simulink model "Simulink_Program_June26 1"  (R2023b)
settings: Solver=VariableStepAuto  StartTime=0.0  StopTime=1  FixedStep=0.001  RelTol=1e-3
libraries: fl_lib x11, nesl_utility x9, ee_lib x7
settings Model: Creator=romul  LastModifiedBy=mcmas

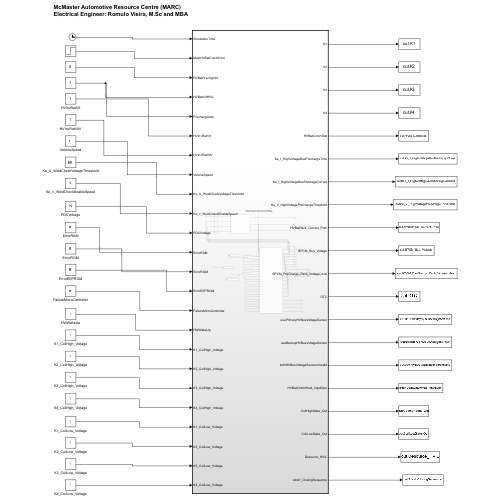
[thumbnail: Simulink's stored preview of the top-level diagram]
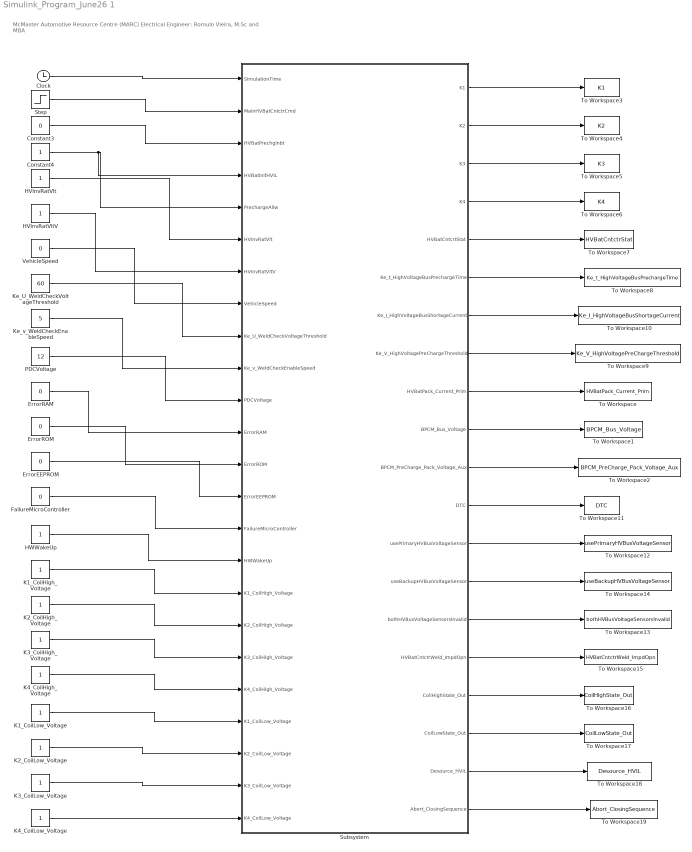
== system Simulink_Program_June26 1 ==
  note: McMaster Automotive Resource Centre (MARC)
      | Electrical Engineer: Romulo Vieira, M.Sc and MBA
  Clock : Clock
  Constant3 : Constant  Value=0
  Constant4 : Constant
  ErrorEEPROM : Constant  Value=0
  ErrorRAM : Constant  Value=0
  ErrorROM : Constant  Value=0
  FailureMicroController : Constant  Value=0
  HVInvRatVlt : Constant
  HVInvRatVltV : Constant
  HWWakeUp : Constant
  K1_CoilHigh_Voltage : Constant
  K1_CoilLow_Voltage : Constant
  K2_CoilHigh_Voltage : Constant
  K2_CoilLow_Voltage : Constant
  K3_CoilHigh_Voltage : Constant
  K3_CoilLow_Voltage : Constant
  K4_CoilHigh_Voltage : Constant
  K4_CoilLow_Voltage : Constant
  Ke_U_WeldCheckVoltageThreshold : Constant  Value=60
  Ke_v_WeldCheckEnableSpeed : Constant  Value=5
  PDCVoltage : Constant  Value=12
  Step : Step  Time=0.5  SampleTime=0.001
  Subsystem : Subsystem  TreatAsAtomicUnit=on
  To Workspace : ToWorkspace  VariableName=HVBatPack_Current_Prim  SampleTime=-1
  To Workspace1 : ToWorkspace  VariableName=BPCM_Bus_Voltage  SampleTime=-1
  To Workspace10 : ToWorkspace  VariableName=Ke_I_HighVoltageBusShortageCurrent  SampleTime=-1
  To Workspace11 : ToWorkspace  VariableName=DTC  SaveFormat=Timeseries  SampleTime=-1
  To Workspace12 : ToWorkspace  VariableName=usePrimaryHVBusVoltageSensor  SaveFormat=Timeseries  SampleTime=-1
  To Workspace13 : ToWorkspace  VariableName=bothHVBusVoltageSensorsInvalid  SaveFormat=Timeseries  SampleTime=-1
  To Workspace14 : ToWorkspace  VariableName=useBackupHVBusVoltageSensor  SaveFormat=Timeseries  SampleTime=-1
  To Workspace15 : ToWorkspace  VariableName=HVBatCntctrWeld_ImpdOpn  SaveFormat=Timeseries  SampleTime=-1
  To Workspace16 : ToWorkspace  VariableName=CoilHighState_Out  SaveFormat=Timeseries  SampleTime=-1
  To Workspace17 : ToWorkspace  VariableName=CoilLowState_Out  SaveFormat=Timeseries  SampleTime=-1
  To Workspace18 : ToWorkspace  VariableName=Desource_HVIL  SaveFormat=Timeseries  SampleTime=-1
  To Workspace19 : ToWorkspace  VariableName=Abort_ClosingSequence  SaveFormat=Timeseries  SampleTime=-1
  To Workspace2 : ToWorkspace  VariableName=BPCM_PreCharge_Pack_Voltage_Aux  SampleTime=-1
  To Workspace3 : ToWorkspace  VariableName=K1  SampleTime=-1
  To Workspace4 : ToWorkspace  VariableName=K2  SampleTime=-1
  To Workspace5 : ToWorkspace  VariableName=K3  SampleTime=-1
  To Workspace6 : ToWorkspace  VariableName=K4  SampleTime=-1
  To Workspace7 : ToWorkspace  VariableName=HVBatCntctrStat  SampleTime=-1
  To Workspace8 : ToWorkspace  VariableName=Ke_t_HighVoltageBusPrechargeTime  SampleTime=-1
  To Workspace9 : ToWorkspace  VariableName=Ke_V_HighVoltagePreChargeThreshold  SampleTime=-1
  VehicleSpeed : Constant  Value=0
  wires:
  Subsystem/3(K3) -> To Workspace5/1
  HVInvRatVltV/1 -> Subsystem/7(HVInvRatVltV)
  Subsystem/15(bothHVBusVoltageSensorsInvalid) -> To Workspace13/1
  Subsystem/6(Ke_t_HighVoltageBusPrechargeTime) -> To Workspace8/1
  HVInvRatVlt/1 -> Subsystem/6(HVInvRatVlt)
  Subsystem/18(CoilLowState_Out) -> To Workspace17/1
  Clock/1 -> Subsystem/1(SimulationTime)
  Constant4/1 -> Subsystem/4(HVBatInitHVIL), Subsystem/5(PrechargeAllw)
  Subsystem/8(Ke_V_HighVoltagePreChargeThreshold) -> To Workspace9/1
  K3_CoilHigh_Voltage/1 -> Subsystem/19(K3_CoilHigh_Voltage)
  Constant3/1 -> Subsystem/3(HVBatPrechgInbt)
  Step/1 -> Subsystem/2(MainHVBatCntctrCmd)
  Ke_U_WeldCheckVoltageThreshold/1 -> Subsystem/9(Ke_U_WeldCheckVoltageThreshold)
  Subsystem/16(HVBatCntctrWeld_ImpdOpn) -> To Workspace15/1
  VehicleSpeed/1 -> Subsystem/8(VehicleSpeed)
  K1_CoilLow_Voltage/1 -> Subsystem/21(K1_CoilLow_Voltage)
  Ke_v_WeldCheckEnableSpeed/1 -> Subsystem/10(Ke_v_WeldCheckEnableSpeed)
  HWWakeUp/1 -> Subsystem/16(HWWakeUp)
  PDCVoltage/1 -> Subsystem/11(PDCVoltage)
  ErrorRAM/1 -> Subsystem/12(ErrorRAM)
  ErrorROM/1 -> Subsystem/13(ErrorROM)
  ErrorEEPROM/1 -> Subsystem/14(ErrorEEPROM)
  FailureMicroController/1 -> Subsystem/15(FailureMicroController)
  Subsystem/1(K1) -> To Workspace3/1
  K1_CoilHigh_Voltage/1 -> Subsystem/17(K1_CoilHigh_Voltage)
  K2_CoilHigh_Voltage/1 -> Subsystem/18(K2_CoilHigh_Voltage)
  K4_CoilHigh_Voltage/1 -> Subsystem/20(K4_CoilHigh_Voltage)
  K2_CoilLow_Voltage/1 -> Subsystem/22(K2_CoilLow_Voltage)
  Subsystem/7(Ke_I_HighVoltageBusShortageCurrent) -> To Workspace10/1
  K3_CoilLow_Voltage/1 -> Subsystem/23(K3_CoilLow_Voltage)
  K4_CoilLow_Voltage/1 -> Subsystem/24(K4_CoilLow_Voltage)
  Subsystem/2(K2) -> To Workspace4/1
  Subsystem/4(K4) -> To Workspace6/1
  Subsystem/5(HVBatCntcrtStat) -> To Workspace7/1
  Subsystem/9(HVBatPack_Current_Prim) -> To Workspace/1
  Subsystem/10(BPCM_Bus_Voltage) -> To Workspace1/1
  Subsystem/14(useBackupHVBusVoltageSensor) -> To Workspace14/1
  Subsystem/12(DTC) -> To Workspace11/1
  Subsystem/11(BPCM_PreCharge_Pack_Voltage_Aux) -> To Workspace2/1
  Subsystem/13(usePrimaryHVBusVoltageSensor) -> To Workspace12/1
  Subsystem/17(CoilHighState_Out) -> To Workspace16/1
  Subsystem/19(Desource_HVIL) -> To Workspace18/1
  Subsystem/20(Abort_ClosingSequence) -> To Workspace19/1

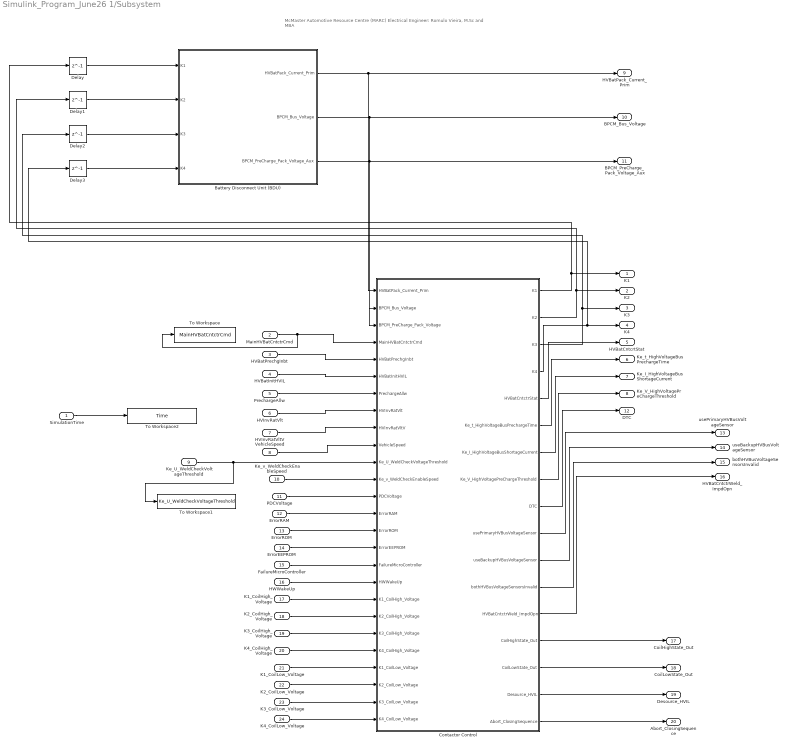
== system Simulink_Program_June26 1/Subsystem ==
  note: McMaster Automotive Resource Centre (MARC)
      | Electrical Engineer: Romulo Vieira, M.Sc and MBA
  SimulationTime : Inport
  MainHVBatCntctrCmd : Inport  Port=2
  HVBatPrechgInbt : Inport  Port=3
  HVBatInitHVIL : Inport  Port=4
  PrechargeAllw : Inport  Port=5
  HVInvRatVlt : Inport  Port=6
  HVInvRatVltV : Inport  Port=7
  VehicleSpeed : Inport  Port=8
  Ke_U_WeldCheckVoltageThreshold : Inport  Port=9
  Ke_v_WeldCheckEnableSpeed : Inport  Port=10
  PDCVoltage : Inport  Port=11
  ErrorRAM : Inport  Port=12
  ErrorROM : Inport  Port=13
  ErrorEEPROM : Inport  Port=14
  FailureMicroController : Inport  Port=15
  HWWakeUp : Inport  Port=16
  K1_CoilHigh_Voltage : Inport  Port=17
  K2_CoilHigh_Voltage : Inport  Port=18
  K3_CoilHigh_Voltage : Inport  Port=19
  K4_CoilHigh_Voltage : Inport  Port=20
  K1_CoilLow_Voltage : Inport  Port=21
  K2_CoilLow_Voltage : Inport  Port=22
  K3_CoilLow_Voltage : Inport  Port=23
  K4_CoilLow_Voltage : Inport  Port=24
  Battery Disconnect Unit (BDU) : Subsystem  TreatAsAtomicUnit=on
  Contactor Control : Subsystem  TreatAsAtomicUnit=on  SystemSampleTime=0.001
  Delay{,1..3} (4 alike) : Delay  DelayLength=1
  To Workspace : ToWorkspace  VariableName=MainHVBatCntctrCmd  SampleTime=-1
  To Workspace1 : ToWorkspace  VariableName=Ke_U_WeldCheckVoltageThreshold  SampleTime=-1
  To Workspace2 : ToWorkspace  VariableName=Time  SampleTime=0.001
  K1 : Outport
  K2 : Outport  Port=2
  K3 : Outport  Port=3
  K4 : Outport  Port=4
  HVBatCntcrtStat : Outport  Port=5
  Ke_t_HighVoltageBusPrechargeTime : Outport  Port=6
  Ke_I_HighVoltageBusShortageCurrent : Outport  Port=7
  Ke_V_HighVoltagePreChargeThreshold : Outport  Port=8
  HVBatPack_Current_Prim : Outport  Port=9
  BPCM_Bus_Voltage : Outport  Port=10
  BPCM_PreCharge_Pack_Voltage_Aux : Outport  Port=11
  DTC : Outport  Port=12
  usePrimaryHVBusVoltageSensor : Outport  Port=13
  useBackupHVBusVoltageSensor : Outport  Port=14
  bothHVBusVoltageSensorsInvalid : Outport  Port=15
  HVBatCntctrWeld_ImpdOpn : Outport  Port=16
  CoilHighState_Out : Outport  Port=17
  CoilLowState_Out : Outport  Port=18
  Desource_HVIL : Outport  Port=19
  Abort_ClosingSequence : Outport  Port=20
  wires:
  Battery Disconnect Unit (BDU)/1(HVBatPack_Current_Prim) -> Contactor Control/1(HVBatPack_Current_Prim), HVBatPack_Current_Prim/1
  Battery Disconnect Unit (BDU)/2(BPCM_Bus_Voltage) -> BPCM_Bus_Voltage/1, Contactor Control/2(BPCM_Bus_Voltage)
  MainHVBatCntctrCmd/1 -> To Workspace/1, Contactor Control/4(MainHVBatCntctrCmd)
  HVBatPrechgInbt/1 -> Contactor Control/5(HVBatPrechgInbt)
  HVBatInitHVIL/1 -> Contactor Control/6(HVBatInitHVIL)
  PrechargeAllw/1 -> Contactor Control/7(PrechargeAllw)
  Contactor Control/1(K1) -> Delay/1, K1/1
  Contactor Control/2(K2) -> Delay1/1, K2/1
  Contactor Control/3(K3) -> Delay2/1, K3/1
  Contactor Control/4(K4) -> Delay3/1, K4/1
  Contactor Control/5(HVBatCntctrStat) -> HVBatCntcrtStat/1
  Contactor Control/6(Ke_t_HighVoltageBusPrechargeTime) -> Ke_t_HighVoltageBusPrechargeTime/1
  Contactor Control/7(Ke_I_HighVoltageBusShortageCurrent) -> Ke_I_HighVoltageBusShortageCurrent/1
  Contactor Control/8(Ke_V_HighVoltagePreChargeThreshold) -> Ke_V_HighVoltagePreChargeThreshold/1
  Battery Disconnect Unit (BDU)/3(BPCM_PreCharge_Pack_Voltage_Aux) -> BPCM_PreCharge_Pack_Voltage_Aux/1, Contactor Control/3(BPCM_PreCharge_Pack_Voltage)
  Delay/1 -> Battery Disconnect Unit (BDU)/1(K1)
  Delay1/1 -> Battery Disconnect Unit (BDU)/2(K2)
  Delay2/1 -> Battery Disconnect Unit (BDU)/3(K3)
  Delay3/1 -> Battery Disconnect Unit (BDU)/4(K4)
  Contactor Control/9(DTC) -> DTC/1
  HVInvRatVlt/1 -> Contactor Control/8(HVInvRatVlt)
  HVInvRatVltV/1 -> Contactor Control/9(HVInvRatVltV)
  Contactor Control/10(usePrimaryHVBusVoltageSensor) -> usePrimaryHVBusVoltageSensor/1
  Contactor Control/11(useBackupHVBusVoltageSensor) -> useBackupHVBusVoltageSensor/1
  Contactor Control/12(bothHVBusVoltageSensorsInvalid) -> bothHVBusVoltageSensorsInvalid/1
  Contactor Control/13(HVBatCntctrWeld_ImpdOpn) -> HVBatCntctrWeld_ImpdOpn/1
  VehicleSpeed/1 -> Contactor Control/10(VehicleSpeed)
  Ke_U_WeldCheckVoltageThreshold/1 -> To Workspace1/1, Contactor Control/11(Ke_U_WeldCheckVoltageThreshold)
  Ke_v_WeldCheckEnableSpeed/1 -> Contactor Control/12(Ke_v_WeldCheckEnableSpeed)
  ErrorRAM/1 -> Contactor Control/14(ErrorRAM)
  ErrorROM/1 -> Contactor Control/15(ErrorROM)
  PDCVoltage/1 -> Contactor Control/13(PDCVoltage)
  FailureMicroController/1 -> Contactor Control/17(FailureMicroController)
  HWWakeUp/1 -> Contactor Control/18(HWWakeUp)
  ErrorEEPROM/1 -> Contactor Control/16(ErrorEEPROM)
  SimulationTime/1 -> To Workspace2/1
  K1_CoilHigh_Voltage/1 -> Contactor Control/19(K1_CoilHigh_Voltage)
  K2_CoilHigh_Voltage/1 -> Contactor Control/20(K2_CoilHigh_Voltage)
  K4_CoilHigh_Voltage/1 -> Contactor Control/22(K4_CoilHigh_Voltage)
  K3_CoilHigh_Voltage/1 -> Contactor Control/21(K3_CoilHigh_Voltage)
  K2_CoilLow_Voltage/1 -> Contactor Control/24(K2_CoilLow_Voltage)
  K1_CoilLow_Voltage/1 -> Contactor Control/23(K1_CoilLow_Voltage)
  K4_CoilLow_Voltage/1 -> Contactor Control/26(K4_CoilLow_Voltage)
  K3_CoilLow_Voltage/1 -> Contactor Control/25(K3_CoilLow_Voltage)
  Contactor Control/14(CoilHighState_Out) -> CoilHighState_Out/1
  Contactor Control/15(CoilLowState_Out) -> CoilLowState_Out/1
  Contactor Control/16(Desource_HVIL) -> Desource_HVIL/1
  Contactor Control/17(Abort_ClosingSequence) -> Abort_ClosingSequence/1

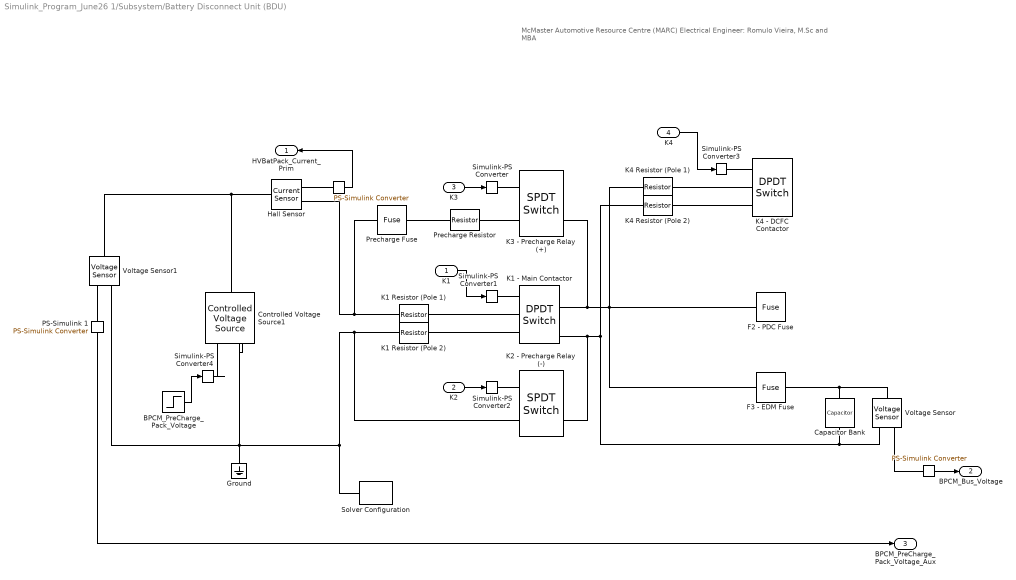
== system Simulink_Program_June26 1/Subsystem/Battery Disconnect Unit (BDU) ==
  note: McMaster Automotive Resource Centre (MARC)
      | Electrical Engineer: Romulo Vieira, M.Sc and MBA
  K1 : Inport
  K2 : Inport  Port=2
  K3 : Inport  Port=3
  K4 : Inport  Port=4
  "   " : nesl_utility/PS-Simulink Converter  PhysicalDomain=network_engine_domain  SubClassName=ps_output  LeftPortType=input  RightPortType=output  PseudoPeriodic=off  Frequencies=[]  VectorFormat=inherit  Unit=inherit  AffineConversion=off
  " " : nesl_utility/PS-Simulink Converter  PhysicalDomain=network_engine_domain  SubClassName=ps_output  LeftPortType=input  RightPortType=output  PseudoPeriodic=off  Frequencies=[]  VectorFormat=inherit  Unit=inherit  AffineConversion=off
  BPCM_PreCharge_Pack_Voltage : Step  Time=0  After=450  SampleTime=0.001
  Capacitor Bank : fl_lib/Electrical/Electrical Elements/Capacitor  c=750e-6 F  r=1e-6 Ohm  g=0 1/Ohm  i_specify=off  i_priority=None  i=0 A  i_nominal_specify=off  i_nominal_unit=A  i_nominal_value=1  v_specify=off  v_priority=None  v=0 V  v_nominal_specify=off  v_nominal_unit=V  v_nominal_value=1  vc_specify=on  vc_priority=High  vc=0 V  vc_nominal_specify=off  vc_nominal_unit=V  vc_nominal_value=1
  Controlled Voltage Source1 : fl_lib/Electrical/Electrical Sources/Controlled Voltage Source
  F2 - PDC Fuse : ee_lib/Switches & Breakers/Fuse  prm=1  I_rated=125 A  melt_margin=1  T_fuse=0 s  I2t=1 A^2*s  I_vec=[1.9, 2, 2.5, 30] A  t_vec=[10000, 1, .3, .001] s  R_closed=0.01 Ohm  G_open=1e-8 1/Ohm  exposemeasurement=ee.enum.exposemeasurement.hidden
      settings: InternalSimscapePortConfiguration="{\"Bottom\":[],\"Left\":[{\"id\":\"p\",\"label\":\"\",\"type\":\"foundation.electrical.electrical\"}],\"Right\":[{\"id\":\"n\",\"label\":\"\",\"type\":\"foundation.electrical.electrical\"}],\"Top\":[]}"
  F3 - EDM Fuse : ee_lib/Switches & Breakers/Fuse  prm=1  I_rated=600 A  melt_margin=1  T_fuse=0 s  I2t=1 A^2*s  I_vec=[1.9, 2, 2.5, 30] A  t_vec=[10000, 1, .3, .001] s  R_closed=0.01 Ohm  G_open=1e-8 1/Ohm  exposemeasurement=ee.enum.exposemeasurement.hidden
      settings: InternalSimscapePortConfiguration="{\"Bottom\":[],\"Left\":[{\"id\":\"p\",\"label\":\"\",\"type\":\"foundation.electrical.electrical\"}],\"Right\":[{\"id\":\"n\",\"label\":\"\",\"type\":\"foundation.electrical.electrical\"}],\"Top\":[]}"
  Ground : fl_lib/Electrical/Electrical Elements/Electrical Reference
  Hall Sensor : fl_lib/Electrical/Electrical Sensors/Current Sensor
  K1 - Main Contactor : ee_lib/Switches & Breakers/DPDT Switch  R_closed=0.01 Ohm  G_open=1e-6 S  Threshold=0.5 V  Width=0 V  model_dynamics=0  t_on=1e-3 s  t_off=1e-3 s  initial_vT=0 V
      settings: InternalSimscapePortConfiguration="{\"Bottom\":[],\"Left\":[{\"id\":\"vT\",\"label\":\"vT\",\"type\":\"input\"},{\"id\":\"p1\",\"label\":\"\",\"type\":\"foundation.electrical.electrical\"},{\"id\":\"p2\",\"label\":\"\",\"type\":\"foundation.electrical.electrical\"}],\"Right\":[{\"id\":\"n11\",\"label\":\"\",\"type\":\"foundation.electrical.electrical\"},{\"id\":\"n12\",\"label\":\"\",\"type\":\"foundation.electrical.electrical\"},{\"id\":\"n21\",\"label\":\"\",\"type\":\"foundation.electrical.electrical\"},{\"id\":\"n22\",\"label\":\"\",\"type\":\"foundation.electrical.electrical\"}],\"Top\":[]}"
  K1 Resistor (Pole 1) : fl_lib/Electrical/Electrical Elements/Resistor  R=0.0003 Ohm  i_specify=off  i_priority=None  i=0 A  i_nominal_specify=off  i_nominal_unit=A  i_nominal_value=1  v_specify=off  v_priority=None  v=0 V  v_nominal_specify=off  v_nominal_unit=V  v_nominal_value=1
  K1 Resistor (Pole 2) : fl_lib/Electrical/Electrical Elements/Resistor  R=0.0003 Ohm  i_specify=off  i_priority=None  i=0 A  i_nominal_specify=off  i_nominal_unit=A  i_nominal_value=1  v_specify=off  v_priority=None  v=0 V  v_nominal_specify=off  v_nominal_unit=V  v_nominal_value=1
  K2 - Precharge Relay (-) : ee_lib/Switches & Breakers/SPDT Switch  R_closed=0.01 Ohm  G_open=1e-6 S  Threshold=0.5 V  Width=0 V  model_dynamics=0  t_on=1e-3 s  t_off=1e-3 s  initial_vT=0 V
  K3 - Precharge Relay (+) : ee_lib/Switches & Breakers/SPDT Switch  R_closed=0.01 Ohm  G_open=1e-6 S  Threshold=0.5 V  Width=0 V  model_dynamics=0  t_on=1e-3 s  t_off=1e-3 s  initial_vT=0 V
  K4 - DCFC Contactor : ee_lib/Switches & Breakers/DPDT Switch  R_closed=0.01 Ohm  G_open=1e-6 S  Threshold=0.5 V  Width=0 V  model_dynamics=0  t_on=1e-3 s  t_off=1e-3 s  initial_vT=0 V
      settings: InternalSimscapePortConfiguration="{\"Bottom\":[],\"Left\":[{\"id\":\"vT\",\"label\":\"vT\",\"type\":\"input\"},{\"id\":\"p1\",\"label\":\"\",\"type\":\"foundation.electrical.electrical\"},{\"id\":\"p2\",\"label\":\"\",\"type\":\"foundation.electrical.electrical\"}],\"Right\":[{\"id\":\"n11\",\"label\":\"\",\"type\":\"foundation.electrical.electrical\"},{\"id\":\"n12\",\"label\":\"\",\"type\":\"foundation.electrical.electrical\"},{\"id\":\"n21\",\"label\":\"\",\"type\":\"foundation.electrical.electrical\"},{\"id\":\"n22\",\"label\":\"\",\"type\":\"foundation.electrical.electrical\"}],\"Top\":[]}"
  K4 Resistor (Pole 1) : fl_lib/Electrical/Electrical Elements/Resistor  R=0.0003 Ohm  i_specify=off  i_priority=None  i=0 A  i_nominal_specify=off  i_nominal_unit=A  i_nominal_value=1  v_specify=off  v_priority=None  v=0 V  v_nominal_specify=off  v_nominal_unit=V  v_nominal_value=1
  K4 Resistor (Pole 2) : fl_lib/Electrical/Electrical Elements/Resistor  R=0.0003 Ohm  i_specify=off  i_priority=None  i=0 A  i_nominal_specify=off  i_nominal_unit=A  i_nominal_value=1  v_specify=off  v_priority=None  v=0 V  v_nominal_specify=off  v_nominal_unit=V  v_nominal_value=1
  PS-Simulink 1 : nesl_utility/PS-Simulink Converter  PhysicalDomain=network_engine_domain  SubClassName=ps_output  LeftPortType=input  RightPortType=output  PseudoPeriodic=off  Frequencies=[]  VectorFormat=inherit  Unit=inherit  AffineConversion=off
  Precharge Fuse : ee_lib/Switches & Breakers/Fuse  prm=1  I_rated=600 A  melt_margin=1  T_fuse=0 s  I2t=1 A^2*s  I_vec=[1.9, 2, 2.5, 30] A  t_vec=[10000, 1, .3, .001] s  R_closed=0.01 Ohm  G_open=1e-8 1/Ohm  exposemeasurement=ee.enum.exposemeasurement.hidden
      settings: InternalSimscapePortConfiguration="{\"Bottom\":[],\"Left\":[{\"id\":\"p\",\"label\":\"\",\"type\":\"foundation.electrical.electrical\"}],\"Right\":[{\"id\":\"n\",\"label\":\"\",\"type\":\"foundation.electrical.electrical\"}],\"Top\":[]}"
  Precharge Resistor : fl_lib/Electrical/Electrical Elements/Resistor  R=25 Ohm  i_specify=off  i_priority=None  i=0 A  i_nominal_specify=off  i_nominal_unit=A  i_nominal_value=1  v_specify=off  v_priority=None  v=0 V  v_nominal_specify=off  v_nominal_unit=V  v_nominal_value=1
  Simulink-PS Converter{,1..3} (4 alike) : nesl_utility/Simulink-PS Converter  PhysicalDomain=network_engine_domain  SubClassName=ps_input  LeftPortType=input  RightPortType=output  PseudoPeriodic=off  Frequencies=[]  NoiseDistribution=none  NoiseParameters=[]  Unit=1  AffineConversion=off  FilteringAndDerivatives=provide  SimscapeFilterOrder=1  InputFilterTimeConstant=0.001  UdotUserProvided=0
  Simulink-PS Converter4 : nesl_utility/Simulink-PS Converter  PhysicalDomain=network_engine_domain  SubClassName=ps_input  LeftPortType=input  RightPortType=output  PseudoPeriodic=off  Frequencies=[]  NoiseDistribution=none  NoiseParameters=[]  Unit=1  AffineConversion=off  FilteringAndDerivatives=filter  SimscapeFilterOrder=1  InputFilterTimeConstant=0.0000001  UdotUserProvided=0
  Solver Configuration : nesl_utility/Solver Configuration  PhysicalDomain=network_engine_domain  SubClassName=solver  LeftPortType=input  RightPortType=generic  Tones=[]  Harmonics=[]  SimulateNoise=off  Profile=off  UseLocalSampling=off  EnableSwitchedLinearOptims=on  FrequencyDomain=off  UseCCode=off  RelTol=0.001  AbsTol=0.001  MinStep=1e-09  ToWorkspace=off  RevertToSquareIcSolve=off  NumHomotopyIterations=100  PhasorMode=off  PhasorModeNumHarmonics=1  ConsistencySolver=NEWTON_XTOL_AFTER_FTOL  IndexReductionMethod=DerivativeReplacement  DoDC=off  ResidualTolerance=1e-09  ConsistencyTolSource=GLOBAL  ConsistencyAbsTol=0.001  ConsistencyRelTol=0.001  ConsistencyTolFactor=0.001  UseLocalSolver=off  LocalSolverChoice=NE_BACKWARD_EULER_ADVANCER  ResolveIndetEquations=on  FunctionEvalNumThread=1  LocalSolverSampleTime=0.001  DoFixedCost=off  MaxNonlinIter=3  MaxModeIter=2  ComputeImpulses=off  ImpulseIterations=2  LinearAlgebra=auto  LinearAlgebraNumThread=0  EquationFormulation=NE_TIME_EF  DelaysMemoryBudget=1024  AutomaticFiltering=on  FilteringTimeConstant=0.001  PartitionStorageMethod=AS_NEEDED  PartitionMemoryBudget=1024  PartitionMethod=ROBUST  MultibodyUseLocalSolver=off  MultibodyLocalSolverChoice=ODE1  MultibodyLocalSolverSampleTime=0.001
  Voltage Sensor : fl_lib/Electrical/Electrical Sensors/Voltage Sensor
  Voltage Sensor1 : fl_lib/Electrical/Electrical Sensors/Voltage Sensor
  HVBatPack_Current_Prim : Outport
  BPCM_Bus_Voltage : Outport  Port=2
  BPCM_PreCharge_Pack_Voltage_Aux : Outport  Port=3
  wires:
  K4/1 -> Simulink-PS Converter3/1
  K3/1 -> Simulink-PS Converter/1
  "   "/1 -> HVBatPack_Current_Prim/1
  K1/1 -> Simulink-PS Converter1/1
  K2/1 -> Simulink-PS Converter2/1
  BPCM_PreCharge_Pack_Voltage/1 -> Simulink-PS Converter4/1
  " "/1 -> BPCM_Bus_Voltage/1
  PS-Simulink 1/1 -> BPCM_PreCharge_Pack_Voltage_Aux/1
  connections:
  K1 Resistor (Pole 2)/LConn1 -- K1 - Main Contactor/LConn3
  Capacitor Bank/LConn1 -- Voltage Sensor/LConn1 -- F3 - EDM Fuse/LConn1
  K2 - Precharge Relay (-)/RConn2 -- K1 - Main Contactor/RConn4 -- Voltage Sensor/RConn2 -- Capacitor Bank/RConn1 -- K4 Resistor (Pole 2)/RConn1
  Hall Sensor/RConn2 -- Precharge Fuse/LConn1 -- K1 Resistor (Pole 1)/RConn1
  K3 - Precharge Relay (+)/RConn2 -- K4 Resistor (Pole 1)/RConn1 -- F2 - PDC Fuse/RConn1 -- F3 - EDM Fuse/RConn1 -- K1 - Main Contactor/RConn2
  Precharge Resistor/LConn1 -- K3 - Precharge Relay (+)/LConn2
  Simulink-PS Converter2/RConn1 -- K2 - Precharge Relay (-)/LConn1
  Precharge Resistor/RConn1 -- Precharge Fuse/RConn1
  Simulink-PS Converter1/RConn1 -- K1 - Main Contactor/LConn1
  Controlled Voltage Source1/LConn1 -- Hall Sensor/LConn1 -- Voltage Sensor1/LConn1
  Simulink-PS Converter/RConn1 -- K3 - Precharge Relay (+)/LConn1
  Voltage Sensor/RConn1 -- " "/LConn1
  K4 - DCFC Contactor/LConn1 -- Simulink-PS Converter3/RConn1
  "   "/LConn1 -- Hall Sensor/RConn1
  Simulink-PS Converter4/RConn1 -- Controlled Voltage Source1/RConn1
  Voltage Sensor1/RConn1 -- PS-Simulink 1/LConn1
  K1 Resistor (Pole 1)/LConn1 -- K1 - Main Contactor/LConn2
  Solver Configuration/RConn1 -- Ground/LConn1 -- Voltage Sensor1/RConn2 -- Controlled Voltage Source1/RConn2 -- K2 - Precharge Relay (-)/LConn2 -- K1 Resistor (Pole 2)/RConn1
  K4 - DCFC Contactor/LConn2 -- K4 Resistor (Pole 1)/LConn1
  K4 Resistor (Pole 2)/LConn1 -- K4 - DCFC Contactor/LConn3

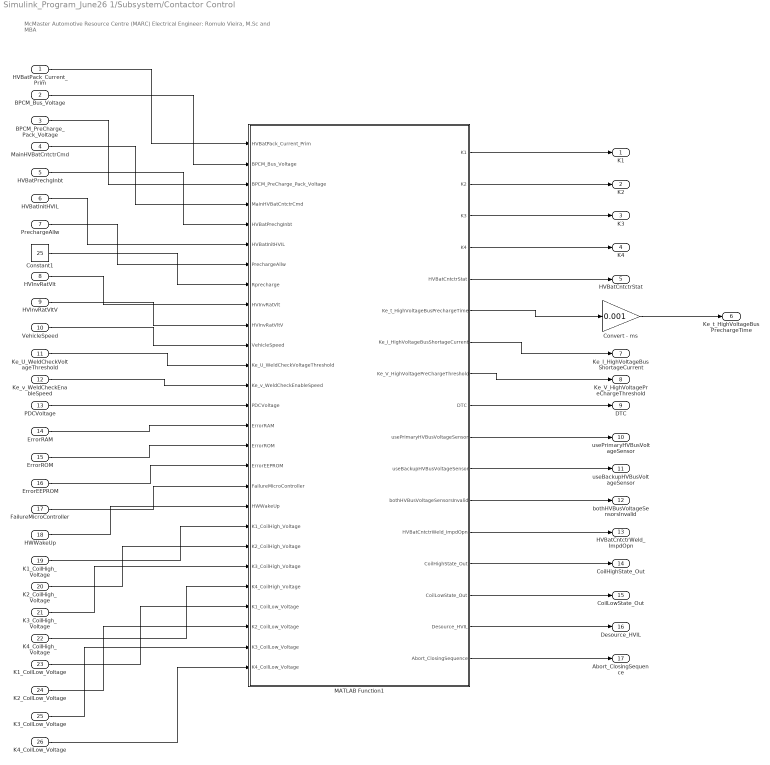
== system Simulink_Program_June26 1/Subsystem/Contactor Control ==
  note: McMaster Automotive Resource Centre (MARC)
      | Electrical Engineer: Romulo Vieira, M.Sc and MBA
  HVBatPack_Current_Prim : Inport
  BPCM_Bus_Voltage : Inport  Port=2
  BPCM_PreCharge_Pack_Voltage : Inport  Port=3
  MainHVBatCntctrCmd : Inport  Port=4
  HVBatPrechgInbt : Inport  Port=5
  HVBatInitHVIL : Inport  Port=6
  PrechargeAllw : Inport  Port=7
  HVInvRatVlt : Inport  Port=8
  HVInvRatVltV : Inport  Port=9
  VehicleSpeed : Inport  Port=10
  Ke_U_WeldCheckVoltageThreshold : Inport  Port=11
  Ke_v_WeldCheckEnableSpeed : Inport  Port=12
  PDCVoltage : Inport  Port=13
  ErrorRAM : Inport  Port=14
  ErrorROM : Inport  Port=15
  ErrorEEPROM : Inport  Port=16
  FailureMicroController : Inport  Port=17
  HWWakeUp : Inport  Port=18
  K1_CoilHigh_Voltage : Inport  Port=19
  K2_CoilHigh_Voltage : Inport  Port=20
  K3_CoilHigh_Voltage : Inport  Port=21
  K4_CoilHigh_Voltage : Inport  Port=22
  K1_CoilLow_Voltage : Inport  Port=23
  K2_CoilLow_Voltage : Inport  Port=24
  K3_CoilLow_Voltage : Inport  Port=25
  K4_CoilLow_Voltage : Inport  Port=26
  Constant1 : Constant  Value=25
  Convert - ms : Gain  Gain=0.001
  MATLAB Function1 : MATLAB Function  SystemSampleTime=0.001
  K1 : Outport
  K2 : Outport  Port=2
  K3 : Outport  Port=3
  K4 : Outport  Port=4
  HVBatCntctrStat : Outport  Port=5
  Ke_t_HighVoltageBusPrechargeTime : Outport  Port=6
  Ke_I_HighVoltageBusShortageCurrent : Outport  Port=7
  Ke_V_HighVoltagePreChargeThreshold : Outport  Port=8
  DTC : Outport  Port=9
  usePrimaryHVBusVoltageSensor : Outport  Port=10
  useBackupHVBusVoltageSensor : Outport  Port=11
  bothHVBusVoltageSensorsInvalid : Outport  Port=12
  HVBatCntctrWeld_ImpdOpn : Outport  Port=13
  CoilHighState_Out : Outport  Port=14
  CoilLowState_Out : Outport  Port=15
  Desource_HVIL : Outport  Port=16
  Abort_ClosingSequence : Outport  Port=17
  wires:
  MATLAB Function1/11(useBackupHVBusVoltageSensor) -> useBackupHVBusVoltageSensor/1
  MATLAB Function1/10(usePrimaryHVBusVoltageSensor) -> usePrimaryHVBusVoltageSensor/1
  HVBatInitHVIL/1 -> MATLAB Function1/6(HVBatInitHVIL)
  MainHVBatCntctrCmd/1 -> MATLAB Function1/4(MainHVBatCntctrCmd)
  MATLAB Function1/5(HVBatCntctrStat) -> HVBatCntctrStat/1
  HVBatPack_Current_Prim/1 -> MATLAB Function1/1(HVBatPack_Current_Prim)
  Constant1/1 -> MATLAB Function1/8(Rprecharge)
  Ke_v_WeldCheckEnableSpeed/1 -> MATLAB Function1/13(Ke_v_WeldCheckEnableSpeed)
  HVInvRatVlt/1 -> MATLAB Function1/9(HVInvRatVlt)
  HVBatPrechgInbt/1 -> MATLAB Function1/5(HVBatPrechgInbt)
  BPCM_PreCharge_Pack_Voltage/1 -> MATLAB Function1/3(BPCM_PreCharge_Pack_Voltage)
  Ke_U_WeldCheckVoltageThreshold/1 -> MATLAB Function1/12(Ke_U_WeldCheckVoltageThreshold)
  BPCM_Bus_Voltage/1 -> MATLAB Function1/2(BPCM_Bus_Voltage)
  PrechargeAllw/1 -> MATLAB Function1/7(PrechargeAllw)
  MATLAB Function1/13(HVBatCntctrWeld_ImpdOpn) -> HVBatCntctrWeld_ImpdOpn/1
  ErrorEEPROM/1 -> MATLAB Function1/17(ErrorEEPROM)
  HVInvRatVltV/1 -> MATLAB Function1/10(HVInvRatVltV)
  MATLAB Function1/9(DTC) -> DTC/1
  ErrorROM/1 -> MATLAB Function1/16(ErrorROM)
  VehicleSpeed/1 -> MATLAB Function1/11(VehicleSpeed)
  MATLAB Function1/4(K4) -> K4/1
  PDCVoltage/1 -> MATLAB Function1/14(PDCVoltage)
  ErrorRAM/1 -> MATLAB Function1/15(ErrorRAM)
  MATLAB Function1/3(K3) -> K3/1
  FailureMicroController/1 -> MATLAB Function1/18(FailureMicroController)
  HWWakeUp/1 -> MATLAB Function1/19(HWWakeUp)
  Convert - ms/1 -> Ke_t_HighVoltageBusPrechargeTime/1
  K1_CoilHigh_Voltage/1 -> MATLAB Function1/20(K1_CoilHigh_Voltage)
  K2_CoilHigh_Voltage/1 -> MATLAB Function1/21(K2_CoilHigh_Voltage)
  K3_CoilHigh_Voltage/1 -> MATLAB Function1/22(K3_CoilHigh_Voltage)
  K4_CoilHigh_Voltage/1 -> MATLAB Function1/23(K4_CoilHigh_Voltage)
  K1_CoilLow_Voltage/1 -> MATLAB Function1/24(K1_CoilLow_Voltage)
  K2_CoilLow_Voltage/1 -> MATLAB Function1/25(K2_CoilLow_Voltage)
  K3_CoilLow_Voltage/1 -> MATLAB Function1/26(K3_CoilLow_Voltage)
  MATLAB Function1/16(Desource_HVIL) -> Desource_HVIL/1
  K4_CoilLow_Voltage/1 -> MATLAB Function1/27(K4_CoilLow_Voltage)
  MATLAB Function1/2(K2) -> K2/1
  MATLAB Function1/1(K1) -> K1/1
  MATLAB Function1/6(Ke_t_HighVoltageBusPrechargeTime) -> Convert - ms/1
  MATLAB Function1/7(Ke_I_HighVoltageBusShortageCurrent) -> Ke_I_HighVoltageBusShortageCurrent/1
  MATLAB Function1/8(Ke_V_HighVoltagePreChargeThreshold) -> Ke_V_HighVoltagePreChargeThreshold/1
  MATLAB Function1/12(bothHVBusVoltageSensorsInvalid) -> bothHVBusVoltageSensorsInvalid/1
  MATLAB Function1/14(CoilHighState_Out) -> CoilHighState_Out/1
  MATLAB Function1/15(CoilLowState_Out) -> CoilLowState_Out/1
  MATLAB Function1/17(Abort_ClosingSequence) -> Abort_ClosingSequence/1

== matlab function Simulink_Program_June26 1/Subsystem/Contactor Control/MATLAB Function1 ==
  data: HVBatPack_Current_Prim input; BPCM_Bus_Voltage input; BPCM_PreCharge_Pack_Voltage input; MainHVBatCntctrCmd input; K1 output; HVBatPrechgInbt input; HVBatInitHVIL input; PrechargeAllw input; K2 output; K3 output; K4 output; HVBatCntctrStat output; Ke_t_HighVoltageBusPrechargeTime output; Ke_I_HighVoltageBusShortageCurrent output; Ke_V_HighVoltagePreChargeThreshold output; Rprecharge input; DTC output; HVInvRatVlt input; HVInvRatVltV input; usePrimaryHVBusVoltageSensor output; useBackupHVBusVoltageSensor output; bothHVBusVoltageSensorsInvalid output; HVBatCntctrWeld_ImpdOpn output; VehicleSpeed input; Ke_U_WeldCheckVoltageThreshold input; Ke_v_WeldCheckEnableSpeed input; PDCVoltage input; ErrorRAM input; ErrorROM input; ErrorEEPROM input; FailureMicroController input; HWWakeUp input; K1_CoilHigh_Voltage input; K2_CoilHigh_Voltage input; K3_CoilHigh_Voltage input; K4_CoilHigh_Voltage input; K1_CoilLow_Voltage input; K2_CoilLow_Voltage input; K3_CoilLow_Voltage input; K4_CoilLow_Voltage input; CoilHighState_Out output; CoilLowState_Out output; Desource_HVIL output; Abort_ClosingSequence output
% McMaster Automotive Resource Centre (MARC)
% Electrical Engineer: Romulo Vieira, M.Sc and MBA - PhD Candidate
function [K1, K2, K3, K4, HVBatCntctrStat, Ke_t_HighVoltageBusPrechargeTime, Ke_I_HighVoltageBusShortageCurrent, Ke_V_HighVoltagePreChargeThreshold, DTC, usePrimaryHVBusVoltageSensor, useBackupHVBusVoltageSensor, bothHVBusVoltageSensorsInvalid, HVBatCntctrWeld_ImpdOpn, CoilHighState_Out, CoilLowState_Out, Desource_HVIL, Abort_ClosingSequence] = prechargeSequencerNoClock( ...
     HVBatPack_Current_Prim, BPCM_Bus_Voltage, BPCM_PreCharge_Pack_Voltage, MainHVBatCntctrCmd, HVBatPrechgInbt, HVBatInitHVIL, PrechargeAllw, Rprecharge, HVInvRatVlt, HVInvRatVltV, VehicleSpeed, Ke_U_WeldCheckVoltageThreshold, Ke_v_WeldCheckEnableSpeed, PDCVoltage, ErrorRAM, ErrorROM, ErrorEEPROM, FailureMicroController, HWWakeUp, K1_CoilHigh_Voltage, K2_CoilHigh_Voltage, K3_CoilHigh_Voltage, K4_CoilHigh_Voltage, K1_CoilLow_Voltage, K2_CoilLow_Voltage, K3_CoilLow_Voltage, K4_CoilLow_Voltage) 

% Input description:
% HVInvRatVlt = Backup HV bus reading 
% HVInvRatVltV = validity of backup HV bus reading                                                                                                                                                                                     
% BPCM_Bus_Voltage = link voltage but is also primary HV bus reading
% MainHVBatCntctrCmd => 0 means open, 1 means close, 2 means fast open
% Removed: InternalHVIL_Valid = validity flag to detect if internal HVIL is passed (last sentence of section I-12)
% Removed: ExternalHVIL_Valid = validity flag to detect if external HVIL is passed (last sentence of section I-12)
% HVBatCntctrStat values and meaning:
% 0: Open
% 1: Precharging
% 2: Closed
% 3: Precharge failed
% 4: Precharge inhibited
% 5: Impending open
% 6: Impact open
% 7: Signal Not Available

% VehicleSpeed = Vehicle's real-time speed
% Ke_U_WeldCheckVoltageThreshold = The minimum HV bus voltage after opening contactors that would indicate a possible weld. This value is set to 60 V in the constant input block.
% Ke_v_WeldCheckEnableSpeed = Maximum vehicle speed at which weld check is allowed to be performed. This value is set to 5 km/h in the constant input block.

%-----------------------------------------------------------
% Purpose: Manage precharge relay and contactor sequence without an external clock
% Controls how the HV bus charges up safely to near pack voltage
% Tracks time window where precharge relays were active
%-----------------------------------------------------------

% Declare persistent variables (retain values across function calls)
persistent I_buffer V_buffer idx Stage HVBatCntctrStat_Aux Ke_idx fill_count prev_PrechargeAllw stage2_count prev_HVBatPack_Current_Prim prev_MainHVBatCntctrCmd prev_HVBatCntctrStat Ke_b_WeldCheckEnabler isWeldFaultLatched weldCheck_retry prev_HWWakeUp dischargeTimer shutdownInProgress CoilHighState CoilLowState

% Declare constants
Buffer_length                      = 100; % Buffer to store 100 ms worth of data (1 ms sample rate in Matlab function)
Ke_V_HighVoltagePreChargeThreshold = 0.99 * BPCM_PreCharge_Pack_Voltage; % Target voltage: 98.5% of pack voltage
Unset_Ke_idx                       = -1; % Marker to indicate target not reached yet
Min_Stage2_Samples                 = 1; % Minimum time (samples) to stay in Stage 2
prechargeTooShortTime              = 20; % Precharge is too short if it's completed within 20 ms of starting
Ke_V_BusSensorFailureThreshold     = 5; % If the primary sensor and auxiliary sensor has more than 5V difference, it means the primary sensors is working fine. It's a calibration constant todetermine whether the primary sensor, i.e., BPCM_Bus_Voltage is providing credible data 
Ke_V_Threshold_HighSide            = 18;  % V (for shorted high) (Section I-16)
Ke_V_Threshold_LowSide             = 2;   % V (for shorted low or open detection) (Section I-16)

% Initialize persistent variables on first call
if isempty(I_buffer)
    I_buffer            = zeros(Buffer_length,1); % Precharge current buffer
    V_buffer            = zeros(Buffer_length,1); % Precharge voltage buffer
    idx                 = 1; % Index for buffers
    Stage               = 0; % Initial internal stage
    HVBatCntctrStat_Aux = 0; % Initial stage for the contactor control
    Ke_idx              = Unset_Ke_idx; % Target voltage not reached yet
    fill_count          = 0; % Counter for Stage 1 samples
    prev_PrechargeAllw  = 0; % Track previous PrechargeAllw
    stage2_count        = 0; % Counter for Stage 2 duration
    prev_HVBatPack_Current_Prim = HVBatPack_Current_Prim; % Initialize previous current sample for derivative calculation
end

if isempty(prev_MainHVBatCntctrCmd)
    prev_MainHVBatCntctrCmd = 0; % keep track of the previous MainHVBatCntctrCmd value (Section I-12 third paragraph to store prev key cycle's value)
end

if isempty(prev_HVBatCntctrStat)
    prev_HVBatCntctrStat = 0; % keep track of the previous HVBatCntctrStat value (Section I-14 first bullet point)
end

if isempty(Ke_b_WeldCheckEnabler)
    Ke_b_WeldCheckEnabler = 1; % Default: enabled
end

if isempty(isWeldFaultLatched)
    isWeldFaultLatched = 0;
end
if isempty(weldCheck_retry)
    weldCheck_retry = 0;
end
if isempty(prev_HWWakeUp)
    prev_HWWakeUp = 0;
end

if isempty(dischargeTimer)
    dischargeTimer = 0; % persistent counter incrementing when shutdown is in progress
end

if isempty(shutdownInProgress)
    shutdownInProgress = 0;
end

if isempty(CoilHighState) || isempty(CoilLowState)
    CoilHighState = zeros(1, 4);
    CoilLowState  = zeros(1, 4);
end

% Default outputs
K1 = 0; K2 = 0; K3 = 0; K4 = 0;
HVBatCntctrStat = HVBatCntctrStat_Aux;

% DTC Values and their meaning
% 0: default (no error)
% 1: Precharging
% 2: Closed
% 3: Precharge failed
% 4: Precharge inhibited
% 5: Impending open
% 6: Impact open
% 7: Signal Not Available
% 8: HV circuit is shorted
% 9: Precharge too long
% 10: Precharge too short
% 11: Forced fast open (Section I-12 second last paragraph)
% 12: Contactor open while commanded closed
% 13: HVIL not valid
% 14: Allow closure in next key cycle (Section I-12 third paragraph)
% 15: Welded contactor has been detected (Section I-13 fourth paragraph)
% 16: Contactor control high side drive circuit shorted high
% 17: Contactor control high side drive circuit shorted low
% 18: Contactor control high side drive circuit open
% 19: Contactor control low side drive circuit shorted high
% 20: Contactor control low side drive circuit shorted low
% 21: Contactor control low side drive circuit open
% 22: At least one contactor is stuck open

DTC                                = 0; % Diagnostic Trouble Code
usePrimaryHVBusVoltageSensor       = 0; % primary HV bus reading validity
useBackupHVBusVoltageSensor        = 0; % backup HV bus reading validity
bothHVBusVoltageSensorsInvalid     = 0; % flag to detect if both sensors' reading is non-credible
HVBatCntctrWeld_ImpdOpn            = 0; % HVBatCntctrWeld_ImpdOpn = Detect if a contactor is welded 

% HVBatCntctrWeld_ImpdOpn values and their meaning
% 0: not welded
% 1: STUCK_CLOSED
% 2: STUCK_OPEN

Desource_HVIL                       = 0; % desource HVIL if stuck open detected (Section I-17)
Abort_ClosingSequence               = 0; % Abort contactor closing if stuck open detected (Section I-17)


switch Stage
    case 0
        % All contactors off
        if MainHVBatCntctrCmd == 1 && HVBatPrechgInbt == 0 && HVBatInitHVIL == 1 && PrechargeAllw == 1
            % Start precharge
            Stage = 1;
            HVBatCntctrStat_Aux = 1;
            I_buffer(:) = 0;
            V_buffer(:) = 0;
            idx = 1;
            Ke_idx = Unset_Ke_idx;
            fill_count = 0;
            stage2_count = 0;
        end

    case 1
        % Precharge relays on
        K1 = 0; K2 = 1; K3 = 1; K4 = 0;

        if fill_count == 0
            % First precharge sample: log initial current from Vpack and V_HVbus = 0
            I_buffer(idx) = BPCM_PreCharge_Pack_Voltage / Rprecharge; % expected initial current at t=0
        else
            % Normal logging
            I_buffer(idx) = HVBatPack_Current_Prim;
        end
        V_buffer(idx) = BPCM_Bus_Voltage;

        % Check if Vtarget first hit
        if Ke_idx == Unset_Ke_idx && BPCM_Bus_Voltage >= Ke_V_HighVoltagePreChargeThreshold
            Ke_idx = fill_count + 1; % Save when Vtarget was first hit
        end

        % Update fill count
        fill_count = fill_count + 1;

        % Increment and wrap index
        idx = idx + 1;
        if idx > Buffer_length
            idx = 1;
        end

        % Evaluate conditions
        maxI = max(I_buffer);

        if Ke_idx ~= Unset_Ke_idx
            delta_samples = Ke_idx;
        else
            delta_samples = fill_count; % in progress
        end

        if Ke_idx ~= Unset_Ke_idx && delta_samples <= Buffer_length && maxI > 10
            % Success → move to Stage 2
            Stage = 2;
            HVBatCntctrStat_Aux = 1;
            stage2_count = 0; % Start counting Stage 2 duration
        elseif fill_count >= Buffer_length
            Stage = 0; % Fail: reset
            HVBatCntctrStat_Aux = 0;
        end

    case 2
        % Main contactor on, precharge relays also on
        K1 = 1; K2 = 0; K3 = 0; K4 = 0;

        % Increment Stage 2 counter
        stage2_count = stage2_count + 1;

        % Check if we've stayed long enough
        if stage2_count >= Min_Stage2_Samples
            Stage = 3;
            HVBatCntctrStat_Aux = 2;
        end

    case 3
        % Stay latched in Stage 3 until PrechargeAllw 0->1 transition
        K1 = 1; K2 = 0; K3 = 0; K4 = 0;

        if prev_PrechargeAllw == 0 && PrechargeAllw == 1
            % Detected re-arm condition
            Stage = 0;
            HVBatCntctrStat_Aux = 0;
            I_buffer(:) = 0;
            V_buffer(:) = 0;
            idx = 1;
            Ke_idx = Unset_Ke_idx;
            fill_count = 0;
            stage2_count = 0;
        end

    otherwise
        % Safety fallback
        K1 = 0; K2 = 0; K3 = 0; K4 = 0;
        Stage = 0;
        HVBatCntctrStat_Aux = 0;
end

HVBatCntctrStat = HVBatCntctrStat_Aux;

% Debug outputs
Ke_t_HighVoltageBusPrechargeTime = Ke_idx;
Ke_I_HighVoltageBusShortageCurrent = max(I_buffer);

if Ke_t_HighVoltageBusPrechargeTime < 0
    Ke_t_HighVoltageBusPrechargeTime = 0;
else
    Ke_t_HighVoltageBusPrechargeTime = Ke_t_HighVoltageBusPrechargeTime + Min_Stage2_Samples;
end

%% Section I-9: Precharge diagnostics
if fill_count > 1
    % Detect bus short based on current threshold and increasing slope
    dt = 0.001; 
    dCurrent_dt = (HVBatPack_Current_Prim - prev_HVBatPack_Current_Prim) / dt;
     
    if HVBatPack_Current_Prim >= Ke_I_HighVoltageBusShortageCurrent && dCurrent_dt >= 0
        DTC = 8;
    end
     
    prev_HVBatPack_Current_Prim = HVBatPack_Current_Prim;
    
    % Detect if precharge is taking too long to complete
    if Ke_t_HighVoltageBusPrechargeTime > Buffer_length && BPCM_Bus_Voltage < Ke_V_HighVoltagePreChargeThreshold
        DTC = 9;
    end
    
    % Detect if precharge is taking too short to complete
    if Ke_t_HighVoltageBusPrechargeTime < prechargeTooShortTime && BPCM_Bus_Voltage >= Ke_V_HighVoltagePreChargeThreshold && V_buffer(1) < 20
        DTC = 10;
    end
end

%% Section I-11: CAN signals associated with precharge
% Check if primary voltage sensor data is credible
if BPCM_Bus_Voltage >= Ke_V_BusSensorFailureThreshold
    usePrimaryHVBusVoltageSensor = 1;
elseif HVInvRatVlt >= Ke_V_BusSensorFailureThreshold && HVInvRatVltV == 1
    useBackupHVBusVoltageSensor = 1;
else 
    bothHVBusVoltageSensorsInvalid = 1;
end

%% Section I-12: Contactors Opening or Prevented from Closing
% Fast open scenario
if MainHVBatCntctrCmd == 2
    K1 = 0;
    K2 = 0;
    K3 = 0;
    K4 = 0;
    HVBatCntctrStat = 0;
    DTC = 11;
end

% Precharge inhibited if conditions are not met
if HVBatInitHVIL ~= 1
    HVBatCntctrStat = 4; % Precharge inhibited
    DTC = 13;
end

if HVBatPrechgInbt ~= 0
    HVBatCntctrStat = 4; % Precharge inhibited
    DTC = 4;
end

% Local variable to track whether precharge is complete
PrechargeComplete = (BPCM_Bus_Voltage >= Ke_V_HighVoltagePreChargeThreshold) && (Stage >= 2);

if MainHVBatCntctrCmd == 1
    if PrechargeComplete
        % Precharge complete => close main and DCFC contactors
        K1 = 1;
        K4 = 1;
        HVBatCntctrStat = 2; % closed
        DTC = 2;
    else
        % Begin precharge
        K2 = 1;
        K3 = 1;
        HVBatCntctrStat = 1; % Precharging
        DTC = 1;
    end          
end

% Detect contactor opening while commanded closed
if (MainHVBatCntctrCmd == 1 && HVBatCntctrStat == 0)
    HVBatCntctrStat = 3; % Precharge Failed
    DTC = 12;
end

% Detect transition from 0 to 1 (new key cycle)
if (prev_MainHVBatCntctrCmd == 0 && MainHVBatCntctrCmd == 1)
    % Allow closure next key cycle if fault gone
    if DTC == 0 && HVBatPrechgInbt == 0
        HVBatCntctrStat = 0; % Ready to retry
        DTC = 14;
    end
end

%% Section I-13 & I-14: Contactor weld check diagnostics & conditions when to perform contactor weld check
% Detect transition from CLOSED (2) to OPEN (0)
if (prev_HVBatCntctrStat == 2 && HVBatCntctrStat == 0)
    % Perform weld check only if all required conditions are true
    if (Ke_b_WeldCheckEnabler == 1 && VehicleSpeed <= Ke_v_WeldCheckEnableSpeed && ~ismember(prev_HVBatCntctrStat, [5, 6, 7]))
        % Check if the bus voltage did not drop. If the bus voltage did not drop, suspect welded contactor.
        % Local variable to track whether weld test is passed (Used in I-13, I-14, I-15)
        weldTest = (BPCM_Bus_Voltage < Ke_U_WeldCheckVoltageThreshold); 
        if weldTest == 0
            HVBatCntctrWeld_ImpdOpn = 1;    % Contactor stuck closed
            HVBatCntctrStat = 5;            % Impending open
            DTC = 15;                       % Weld DTC
        end
    end
end

%% Section I-15: Conditions to Interrupt Contactor Weld Check

% Interrupt conditions — immediately abort the weld check
weldCheckBlocked = (PDCVoltage < 12 || ErrorRAM || ErrorROM || ErrorEEPROM || FailureMicroController || (HWWakeUp == 1 && prev_HWWakeUp == 0));

% Check if weld check is enabled
if Ke_b_WeldCheckEnabler == 1 && ~weldCheckBlocked

    % Detect shutdown start: contactors go from CLOSED to OPEN
    shutdownStarted = (prev_HVBatCntctrStat == 2) && (HVBatCntctrStat == 0);

    % Parameters for discharge timing
    T_discharge_ms = 1000;          % 1000 ms discharge wait
    T_sample = 0.001;               % 1 ms simulation timestep
    T_discharge_samples = T_discharge_ms / (T_sample * 1000);  % 1000 samples

    % Local variable to track whether weld test is passed (Used in I-13, I-14, I-15)
    weldTest = (BPCM_Bus_Voltage < Ke_U_WeldCheckVoltageThreshold); 
    % On shutdown start and failed weld test, begin discharge phase
    if shutdownStarted && weldTest == 0
        shutdownInProgress = 1;  % Mark shutdown process active
        dischargeTimer = 0;      % Reset timer
    end

    % While in shutdown, count discharge time
    if shutdownInProgress == 1
        dischargeTimer = dischargeTimer + 1;

        if dischargeTimer >= T_discharge_samples
            if weldTest == 1
                weldCheck_retry = 0;  % retry passed
            else
                weldCheck_retry = 1;  % retry failed → try again at wake-up
            end
            shutdownInProgress = 0;   % Discharge phase complete
            dischargeTimer = 0;
        end
    end

    % On wake-up: retry weld test if shutdown retry failed
    if HWWakeUp == 1 && weldCheck_retry == 1
        if weldTest ~= 1
            isWeldFaultLatched = 1;
            HVBatCntctrWeld_ImpdOpn = 1;
        end
        weldCheck_retry = 0;
    end
end

% Set DTC if weld fault latched
if isWeldFaultLatched == 1
    DTC = 15;
end

%% Section I-16: Contactor Control Circuit Diagnostic

% Define coil names
coilNames = {'K1', 'K2', 'K3', 'K4'};
numberOfCoils = length(coilNames);
K = [K1, K2, K3, K4];
CoilHigh_V = [K1_CoilHigh_Voltage, K2_CoilHigh_Voltage, K3_CoilHigh_Voltage, K4_CoilHigh_Voltage];
CoilLow_V  = [K1_CoilLow_Voltage,  K2_CoilLow_Voltage,  K3_CoilLow_Voltage,  K4_CoilLow_Voltage];

% Loop through each coil
for i = 1:numberOfCoils
    % Determine which contactor is energized
    if K(i) == 1
        % High side drive diagnostics
        if CoilHigh_V(i) > Ke_V_Threshold_HighSide
            CoilHighState(i) = 2; % SHORTED_HIGH
            DTC = 16; % High side shorted high
        elseif CoilHigh_V(i) < Ke_V_Threshold_LowSide
            CoilHighState(i) = 1; % SHORTED_LOW
            DTC = 17; % High side shorted low
        elseif isnan(CoilHigh_V(i)) || isinf(CoilHigh_V(i)) 
            CoilHighState(i) = 3; % OPEN
            DTC = 18; % High side open
        else
            CoilHighState(i) = 0; % NORMAL
        end
    elseif K(i) == 0
        if CoilLow_V(i) > Ke_V_Threshold_HighSide
            CoilLowState(i) = 2; % SHORTED_HIGH
            DTC = 19; % Low side shorted high
        elseif CoilLow_V(i) < Ke_V_Threshold_LowSide
            CoilLowState(i) = 1; % SHORTED_LOW
            DTC = 20; % Low side shorted low
        elseif isnan(CoilLow_V(i)) || isinf(CoilLow_V(i)) 
            CoilLowState(i) = 3; % OPEN
            DTC = 21; % Low side open
        else
            CoilLowState(i) = 0; % NORMAL
        end    
    end
end

% Output to plot
CoilHighState_Out = CoilHighState; 
CoilLowState_Out = CoilLowState;

%% I-17: Contactor Stuck Open Diagnostics
% Initialize internal per-contactor stuck open vector
HVBatCntctrWeld_ImpdOpnVec = zeros(1, numberOfCoils);

% Internal status flag
ContactorStuckOpen_Flag  = 0;

if MainHVBatCntctrCmd == 1
    % Loop through each coil
    for i = 1:numberOfCoils
        if HVBatCntctrStat ~= 2 % Not in closed state
            HVBatCntctrWeld_ImpdOpnVec(i) = 2;
            ContactorStuckOpen_Flag = 1;
        else
            HVBatCntctrWeld_ImpdOpnVec(i) = 0;
        end
    end

    if ContactorStuckOpen_Flag == 1
        DTC = 22;
        Desource_HVIL = 1;
        Abort_ClosingSequence = 1;
    else
        DTC = 0;
        Desource_HVIL = 0;
        Abort_ClosingSequence = 0;
    end
else
    % No close command - safe defaults
    DTC = 0;
    Desource_HVIL = 0;
    Abort_ClosingSequence = 0;
end

if ContactorStuckOpen_Flag == 1
    HVBatCntctrWeld_ImpdOpn = 2;
else
    HVBatCntctrWeld_ImpdOpn = 0;
end

%% Update prev_PrechargeAllw for edge detection
prev_PrechargeAllw = PrechargeAllw;

% Update prev_MainHVBatCntctrCmd
prev_MainHVBatCntctrCmd = MainHVBatCntctrCmd;

% Update prev_HVBatCntctrStat
prev_HVBatCntctrStat = HVBatCntctrStat;

% Update prev_HWWakeUp
prev_HWWakeUp = HWWakeUp;

end
